simulink model "V_gamma"  (R2018b)
settings: Solver=VariableStepAuto  StartTime=0.0  StopTime=10.0  RelTol=1e-3
undefined symbols (not defined in the file): r_bPGamR
settings Model: Creator=rache  LastModifiedBy=rache

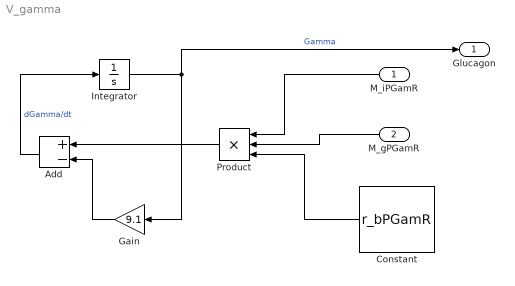
== system V_gamma ==
  M_iPGamR : Inport
  M_gPGamR : Inport  Port=2
  Add : Sum  Inputs=+-
  Constant : Constant  Value=r_bPGamR
  Gain : Gain  Gain=9.1
  Integrator : Integrator
  Product : Product  Inputs=3
  Glucagon : Outport
  wires:
  Add/1 -> Integrator/1  "dGamma/dt"
  Constant/1 -> Product/3
  M_gPGamR/1 -> Product/2
  M_iPGamR/1 -> Product/1
  Product/1 -> Add/1
  Integrator/1 -> Glucagon/1, Gain/1  "Gamma"
  Gain/1 -> Add/2
